simulink model "flywheel_simscape_model"  (R2021a)
settings: Solver=FixedStepAuto  StartTime=0.0  StopTime=2.5  FixedStep=0.01  RelTol=1e-3  AbsTol=1e-3
libraries: fl_lib x10, nesl_utility x4, ee_lib x1
settings Model: Creator=Cameron  LastModifiedBy=elissaito
settings SolverCC: AutoScaleAbsTol=off  AlgebraicLoopSolver=TrustRegion
settings DebuggingCC: SymbolicDimsDataTypeCodeGenerationDiagnostic=none  SFMachineParentedDataDiag=warning
settings SFSimCC: CustomCodeUndefinedFunction=UseInterfaceOnly
settings SimscapeCC: SimscapeLogType=all  SimscapeLogSimulationStatistics=on  SimscapeLogDataHistory=10000

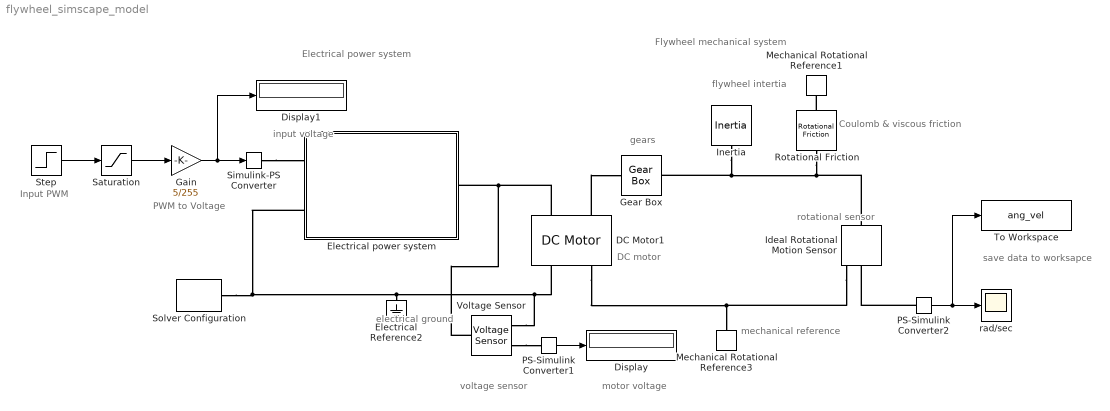
== system flywheel_simscape_model ==
  note: PWM to Voltage
  note: Input PWM
  note: mechanical
      | reference
  note: gears
  note: DC motor
  note: rotational
      | sensor
  note: Coulomb &
      | viscous friction
  note: flywheel
      | intertia
  note: electrical
      | ground
  note: voltage sensor
  note: motor voltage
  note: input voltage
  note: save data to worksapce
  note: Flywheel mechanical system
  note: Electrical power system
  DC Motor1 : ee_lib/Electromechanical/Brushed Motors/DC Motor  field_option=ee.enum.field_option.pm  Rf=100 Ohm  Lf=1 H  Laf=0.15 H  If0=0 A  parameterization=ee.enum.dcparam_option.circuit_param  Ra=3.2 Ohm  La=0.001 mH  emf_or_torque=ee.enum.emf_or_torque.kv  Kv=0.0075 V/(rad/s)  Ki=30.2 mN*m/A  T_stall=0.24e-3 N*m  w_max=4000 rpm  w_rated=2500 rpm  P_rated=10 W  V_rated=12 V  J=25 g*cm^2  lam_param=ee.enum.lam_param.current  lam=1e-6 N*m/(rad/s)  i_noload=140 mA  V_i_noload=12 V  speed0=0 rad/s  enable_fault_armature=ee.enum.faults.faultEnable.no  rev_faulted=1 / 3  G_faulted_armature=1e-5 S  fault_trigger_armature=ee.enum.faults.faultTrigger.temporal  t_fault_armature=1 s  max_permissible_current_armature=inf A  t_fail_on_current_armature=1 s  enable_fault_field=ee.enum.faults.faultEnable.no  G_faulted_field=1e-5 S  fault_trigger_field=ee.enum.faults.faultTrigger.temporal  t_fault_field=1 s  max_permissible_current_field=inf A  t_fail_on_current_field=1 s  fault_action=ee.enum.faults.faultAction.none  alpha=3.93e-3 1/K  Tmeas=25 degC  thermal_mass=100 J/K  initial_temperature=25 degC
  Display : Display
  Display1 : Display
  Electrical Reference2 : fl_lib/Electrical/Electrical Elements/Electrical Reference
  Electrical power system : Subsystem
  Gain : Gain  Gain=5/255
  Gear Box : fl_lib/Mechanical/Mechanisms/Gear Box  ratio=34  t_in_specify=off  t_in_priority=None  t_in=0 N*m  t_in_nominal_specify=off  t_in_nominal_unit=N*m  t_in_nominal_value=1  t_out_specify=off  t_out_priority=None  t_out=0 N*m  t_out_nominal_specify=off  t_out_nominal_unit=N*m  t_out_nominal_value=1
  Ideal Rotational Motion Sensor : fl_lib/Mechanical/Mechanical Sensors/Ideal Rotational Motion Sensor  wrap_angle=simscape.enum.onoff.off  offset=0 rad
  Inertia : fl_lib/Mechanical/Rotational Elements/Inertia  inertia=1.47*10^-4 kg*m^2  num_ports=foundation.enum.numPorts2.one  w_specify=off  w_priority=High  w=0 rad/s  w_nominal_specify=off  w_nominal_unit=rad/s  w_nominal_value=1  t_specify=on  t_priority=Low  t=0 N*m  t_nominal_specify=off  t_nominal_unit=N*m  t_nominal_value=1
  Mechanical Rotational Reference1 : fl_lib/Mechanical/Rotational Elements/Mechanical Rotational Reference
  Mechanical Rotational Reference3 : fl_lib/Mechanical/Rotational Elements/Mechanical Rotational Reference
  PS-Simulink Converter1 : nesl_utility/PS-Simulink Converter  PhysicalDomain=network_engine_domain  SubClassName=ps_output  LeftPortType=input  RightPortType=output  PseudoPeriodic=off  Frequencies=[]  Unit=V  AffineConversion=off
      settings: SourceProductBaseCode=PW,SS
  PS-Simulink Converter2 : nesl_utility/PS-Simulink Converter  PhysicalDomain=network_engine_domain  SubClassName=ps_output  LeftPortType=input  RightPortType=output  PseudoPeriodic=off  Frequencies=[]  Unit=rad/s  AffineConversion=off
      settings: SourceProductBaseCode=PW,SS
  Rotational Friction : fl_lib/Mechanical/Rotational Elements/Rotational Friction  brkwy_trq=0.001 N*m  brkwy_vel=0.01 rad/s  Col_trq=0.001 N*m  visc_coef=0.00096 N*m/(rad/s)  w_specify=on  w_priority=Low  w=0 rad/s  w_nominal_specify=off  w_nominal_unit=rad/s  w_nominal_value=1  t_specify=on  t_priority=Low  t=0 N*m  t_nominal_specify=off  t_nominal_unit=N*m  t_nominal_value=1
  Saturation : Saturate  UpperLimit=255  LowerLimit=-255
  Simulink-PS Converter : nesl_utility/Simulink-PS Converter  PhysicalDomain=network_engine_domain  SubClassName=ps_input  LeftPortType=input  RightPortType=output  PseudoPeriodic=off  Frequencies=[]  NoiseDistribution=none  NoiseParameters=[]  Unit=1  AffineConversion=off  FilteringAndDerivatives=provide  SimscapeFilterOrder=1  InputFilterTimeConstant=0.001  UdotUserProvided=0
      settings: SourceProductBaseCode=PW,SS
  Solver Configuration : nesl_utility/Solver Configuration  PhysicalDomain=network_engine_domain  SubClassName=solver  LeftPortType=input  RightPortType=generic  Tones=[]  Harmonics=[]  SimulateNoise=off  Profile=off  UseLocalSampling=off  EnableSwitchedLinearOptims=on  FrequencyDomain=off  UseCCode=off  RelTol=0.001  AbsTol=1e-06  MinStep=1e-09  ToWorkspace=off  RevertToSquareIcSolve=off  NumHomotopyIterations=100  PhasorMode=off  PhasorModeNumHarmonics=1  DoDC=off  ResidualTolerance=1e-09  UseLocalSolver=off  LocalSolverChoice=NE_BACKWARD_EULER_ADVANCER  LocalSolverSampleTime=0.001  DoFixedCost=off  MaxNonlinIter=3  MaxModeIter=2  ComputeImpulses=off  ImpulseIterations=2  LinearAlgebra=auto  EquationFormulation=NE_TIME_EF  DelaysMemoryBudget=1024  AutomaticFiltering=on  FilteringTimeConstant=0.001  PartitionStorageMethod=AS_NEEDED  PartitionMemoryBudget=1024  PartitionMethod=FAST
      settings: SourceProductBaseCode=PW,SS
  Step : Step  Time=0  After=150  SampleTime=0
  To Workspace : ToWorkspace  VariableName=ang_vel  SaveFormat=Timeseries  SampleTime=-1
  Voltage Sensor : fl_lib/Electrical/Electrical Sensors/Voltage Sensor
  rad/sec : Scope
  wires:
  PS-Simulink Converter2/1 -> To Workspace/1, rad/sec/1
  Gain/1 -> Display1/1, Simulink-PS Converter/1
  Step/1 -> Saturation/1
  Saturation/1 -> Gain/1
  PS-Simulink Converter1/1 -> Display/1
  connections:
  Electrical power system/LConn2 -- Solver Configuration/RConn1 -- Electrical Reference2/LConn1 -- Voltage Sensor/RConn2 -- DC Motor1/RConn1
  PS-Simulink Converter2/LConn1 -- Ideal Rotational Motion Sensor/RConn2
  DC Motor1/LConn2 -- Gear Box/LConn1
  Rotational Friction/LConn1 -- Mechanical Rotational Reference1/LConn1
  DC Motor1/RConn2 -- Mechanical Rotational Reference3/LConn1 -- Ideal Rotational Motion Sensor/RConn1
  Simulink-PS Converter/RConn1 -- Electrical power system/LConn1
  DC Motor1/LConn1 -- Voltage Sensor/LConn1 -- Electrical power system/RConn1
  Inertia/LConn1 -- Gear Box/RConn1 -- Ideal Rotational Motion Sensor/LConn1 -- Rotational Friction/RConn1
  Voltage Sensor/RConn1 -- PS-Simulink Converter1/LConn1

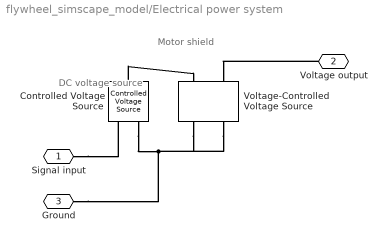
== system flywheel_simscape_model/Electrical power system ==
  note: Motor shield
  note: DC voltage
      | source
  Controlled Voltage Source : fl_lib/Electrical/Electrical Sources/Controlled Voltage Source
  Voltage-Controlled Voltage Source : fl_lib/Electrical/Electrical Sources/Voltage-Controlled Voltage Source  K=12/5  v1_specify=off  v1_priority=None  v1=0 V  v1_nominal_specify=off  v1_nominal_unit=V  v1_nominal_value=1  v2_specify=off  v2_priority=None  v2=0 V  v2_nominal_specify=off  v2_nominal_unit=V  v2_nominal_value=1
      settings: SourceProductBaseCode=SS  InternalSimscapePortConfiguration="{\"Bottom\":[],\"Left\":[{\"id\":\"p1\",\"label\":\"+\",\"type\":\"foundation.electrical.electrical\"},{\"id\":\"p2\",\"label\":\"+\",\"type\":\"foundation.electrical.electrical\"}],\"Right\":[{\"id\":\"n1\",\"label\":\"-\",\"type\":\"foundation.electrical.electrical\"},{\"id\":\"n2\",\"label\":\"-\",\"type\":\"foundation.electrical.electrical\"}],\"Top\":[]}"
  Signal input : PMIOPort  Side=Left
  Voltage output : PMIOPort  Port=2  Side=Right
  Ground : PMIOPort  Port=3  Side=Left
  connections:
  Controlled Voltage Source/RConn2 -- Voltage-Controlled Voltage Source/RConn2 -- Voltage-Controlled Voltage Source/RConn1 -- Ground/RConn1
  Signal input/RConn1 -- Controlled Voltage Source/RConn1
  Controlled Voltage Source/LConn1 -- Voltage-Controlled Voltage Source/LConn1
  Voltage output/RConn1 -- Voltage-Controlled Voltage Source/LConn2
